simulink library "Enrg_conv_El_to_Mec_zfCetrax"  (R2016a)
settings: Solver=ode1  StartTime=0.0  StopTime=Inf  FixedStep=0.001  RelTol=1e-3
undefined symbols (not defined in the file): drvEmot_RefTqeMOT, FirstDrivenAxle_FirstDrivenAxleNoOfEmot, FirstDrivenAxleNoOfEmot, FMIKit, mec_fRollCoeffOverall, mec_iDiffAxle, mec_massVehicle_kg, mec_rWheelDriven, RefTqeMOT, SecondDrivenAxle_SecondDrivenAxleNoOfEmot, SecondDrivenAxleNoOfEmot
libraries: simulink_extras x3, Enrg_conv_El_to_Mec_zfCetrax x3
(part 3 of 3)

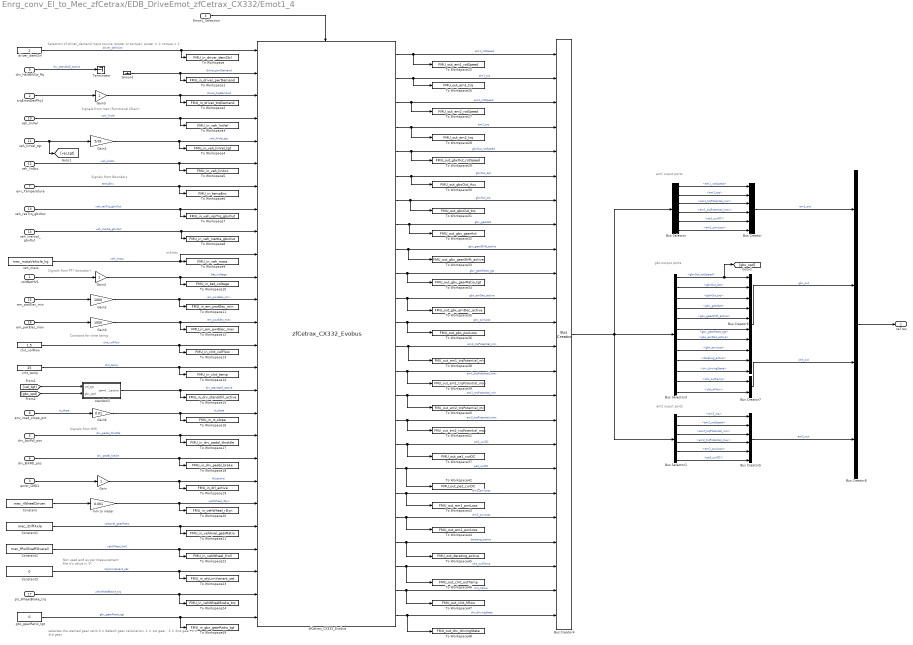
== system Enrg_conv_El_to_Mec_zfCetrax/EDB_DriveEmot_zfCetrax_CX332/Emot1_4 ==
  note: em1 ouput ports
  note: Selection of driver_demand input source (power or torque). power = 1; torque = 2
  note: Signals from Boundary
  note: Signals from HMI
  note: Signals from mec (Functional Chain)
  note: Constant for time being
  note: Signals from PTI (actuator)
  note: em2 ouput ports
  note: gbx output ports
  note: Not used and as per
      | measurement file it's value is '0'
  note: m3/sec
  note: selectes the wanted gear ratio
      | 0 = default gear calculation, 1 = 1st gear , 2 = 2nd gear, 3 = 3rd gear
  voltBatHV1 : Inport
  trqEmotDesPhy1 : Inport  Port=2
  emot_CMD1 : Inport  Port=3
  Emot1_Selection : Inport  Port=4
  drv_AccPdl_pos : Inport  Port=5
  drv_BrkPdl_pos : Inport  Port=6
  env_Temperature : Inport  Port=7
  env_road_slope_pct : Inport  Port=8
  drv_HaltBrkSw_Rq : Inport  Port=9
  veh_linVel : Inport  Port=10
  veh_linVel_tgt : Inport  Port=11
  veh_linAcc : Inport  Port=12
  veh_resTrq_gbxOut : Inport  Port=13
  veh_inertial_gbxOut : Inport  Port=14
  em_pwrElec_min : Inport  Port=15
  em_pwrElec_max : Inport  Port=16
  pti_WheelBrake_trq : Inport  Port=17
  Bus Creator : BusCreator  Inputs=6
  Bus Creator4 : BusCreator  Inputs=24
  Bus Creator5 : BusCreator  Inputs=6
  Bus Creator6 : BusCreator  Inputs=10
  Bus Creator7 : BusCreator  Inputs=2
  Bus Creator8 : BusCreator  Inputs=4
  Bus Selector : BusSelector  OutputSignals=em1_rotSpeed,em1_trq,em1_trqPotential_min,em1_trqPotential_max,pe1_curDC,em1_pwrLoss
  Bus Selector1 : BusSelector  OutputSignals=em2_trq,em2_rotSpeed,em2_trqPotential_min,em2_trqPotential_max,em2_pwrLoss,pe2_curDC
  Bus Selector3 : BusSelector  OutputSignals=gbxOut_rotSpeed,gbxOut_Acc,gbxOut_trq,gbx_gearAct,gbx_gearShift_active,gbx_gearRatio_tgt,gbx_emDec_active,gbx_pwrLoss,derating_active,drv_drivingState,clnt_outTemp,clnt_hFlow
  Constant : Constant  Value=mec_rWheelDriven
  Constant1 : Constant  Value=mec_iDiffAxle
  Constant2 : Constant  Value=mec_fRollCoeffOverall
  Constant3 : Constant  Value=0
  Gain : Gain
  Gain1 : Gain  Gain=5/18
  Gain2 : Gain  Gain=1000
  Gain3 : Gain  Gain=1000
  Gain4 : Gain
  Gain5 : Gain
  Gain6 : Gain  Gain=0.01
  Ground : Ground
  Terminator : Terminator
  To Workspace : ToWorkspace  VariableName=FMU_in_driver_demCtrl  SampleTime=-1
      settings: Save2DSignal=2-D array (concatenate along first dimension)
  To Workspace1 : ToWorkspace  VariableName=FMU_in_driver_pwrDemand  SampleTime=-1
      settings: Save2DSignal=2-D array (concatenate along first dimension)
  To Workspace10 : ToWorkspace  VariableName=FMU_in_bat_voltage  SampleTime=-1
      settings: Save2DSignal=2-D array (concatenate along first dimension)
  To Workspace11 : ToWorkspace  VariableName=FMU_in_em_pwrElec_min  SampleTime=-1
      settings: Save2DSignal=2-D array (concatenate along first dimension)
  To Workspace12 : ToWorkspace  VariableName=FMU_in_em_pwrElec_max  SampleTime=-1
      settings: Save2DSignal=2-D array (concatenate along first dimension)
  To Workspace13 : ToWorkspace  VariableName=FMU_in_clnt_volFlow  SampleTime=-1
      settings: Save2DSignal=2-D array (concatenate along first dimension)
  To Workspace14 : ToWorkspace  VariableName=FMU_in_clnt_temp  SampleTime=-1
      settings: Save2DSignal=2-D array (concatenate along first dimension)
  To Workspace15 : ToWorkspace  VariableName=FMU_in_drv_standstill_active  SampleTime=-1
      settings: Save2DSignal=2-D array (concatenate along first dimension)
  To Workspace16 : ToWorkspace  VariableName=FMU_in_rt_slope  SampleTime=-1
      settings: Save2DSignal=2-D array (concatenate along first dimension)
  To Workspace17 : ToWorkspace  VariableName=FMU_in_drv_pedal_throttle  SampleTime=-1
      settings: Save2DSignal=2-D array (concatenate along first dimension)
  To Workspace18 : ToWorkspace  VariableName=FMU_in_drv_pedal_brake  SampleTime=-1
      settings: Save2DSignal=2-D array (concatenate along first dimension)
  To Workspace19 : ToWorkspace  VariableName=FMU_in_drl_active  SampleTime=-1
      settings: Save2DSignal=2-D array (concatenate along first dimension)
  To Workspace2 : ToWorkspace  VariableName=FMU_in_driver_trqDemand  SampleTime=-1
      settings: Save2DSignal=2-D array (concatenate along first dimension)
  To Workspace20 : ToWorkspace  VariableName=FMU_in_vehWheel_rDyn  SampleTime=-1
      settings: Save2DSignal=2-D array (concatenate along first dimension)
  To Workspace21 : ToWorkspace  VariableName=FMU_in_vehAxel_gearRatio  SampleTime=-1
      settings: Save2DSignal=2-D array (concatenate along first dimension)
  To Workspace22 : ToWorkspace  VariableName=FMU_in_vehWheel_froll  SampleTime=-1
      settings: Save2DSignal=2-D array (concatenate along first dimension)
  To Workspace23 : ToWorkspace  VariableName=FMU_in_styLimVariant_set  SampleTime=-1
      settings: Save2DSignal=2-D array (concatenate along first dimension)
  To Workspace24 : ToWorkspace  VariableName=FMU_in_vehWheelBrake_trq  SampleTime=-1
      settings: Save2DSignal=2-D array (concatenate along first dimension)
  To Workspace25 : ToWorkspace  VariableName=FMU_out_em1_rotSpeed  SampleTime=-1
      settings: Save2DSignal=2-D array (concatenate along first dimension)
  To Workspace26 : ToWorkspace  VariableName=FMU_out_em1_trq  SampleTime=-1
      settings: Save2DSignal=2-D array (concatenate along first dimension)
  To Workspace27 : ToWorkspace  VariableName=FMU_out_em2_rotSpeed  SampleTime=-1
      settings: Save2DSignal=2-D array (concatenate along first dimension)
  To Workspace28 : ToWorkspace  VariableName=FMU_out_em2_trq  SampleTime=-1
      settings: Save2DSignal=2-D array (concatenate along first dimension)
  To Workspace29 : ToWorkspace  VariableName=FMU_out_gbxOut_rotSpeed  SampleTime=-1
      settings: Save2DSignal=2-D array (concatenate along first dimension)
  To Workspace3 : ToWorkspace  VariableName=FMU_in_veh_linVel  SampleTime=-1
      settings: Save2DSignal=2-D array (concatenate along first dimension)
  To Workspace30 : ToWorkspace  VariableName=FMU_out_gbxOut_Acc  SampleTime=-1
      settings: Save2DSignal=2-D array (concatenate along first dimension)
  To Workspace31 : ToWorkspace  VariableName=FMU_out_gbxOut_trq  SampleTime=-1
      settings: Save2DSignal=2-D array (concatenate along first dimension)
  To Workspace32 : ToWorkspace  VariableName=FMU_out_gbx_gearAct  SampleTime=-1
      settings: Save2DSignal=2-D array (concatenate along first dimension)
  To Workspace33 : ToWorkspace  VariableName=FMU_out_gbx_gearShift_active  SampleTime=-1
      settings: Save2DSignal=2-D array (concatenate along first dimension)
  To Workspace34 : ToWorkspace  VariableName=FMU_out_gbx_gearRatio_tgt  SampleTime=-1
      settings: Save2DSignal=2-D array (concatenate along first dimension)
  To Workspace35 : ToWorkspace  VariableName=FMU_out_gbx_emDec_active  SampleTime=-1
      settings: Save2DSignal=2-D array (concatenate along first dimension)
  To Workspace36 : ToWorkspace  VariableName=FMU_out_gbx_pwrLoss  SampleTime=-1
      settings: Save2DSignal=2-D array (concatenate along first dimension)
  To Workspace37 : ToWorkspace  VariableName=FMU_out_pe1_curDC  SampleTime=-1
      settings: Save2DSignal=2-D array (concatenate along first dimension)
  To Workspace38 : ToWorkspace  VariableName=FMU_out_em1_trqPotential_min  SampleTime=-1
      settings: Save2DSignal=2-D array (concatenate along first dimension)
  To Workspace39 : ToWorkspace  VariableName=FMU_out_em1_trqPotential_max  SampleTime=-1
      settings: Save2DSignal=2-D array (concatenate along first dimension)
  To Workspace4 : ToWorkspace  VariableName=FMU_in_veh_linVel_tgt  SampleTime=-1
      settings: Save2DSignal=2-D array (concatenate along first dimension)
  To Workspace40 : ToWorkspace  VariableName=FMU_out_em2_trqPotential_min  SampleTime=-1
      settings: Save2DSignal=2-D array (concatenate along first dimension)
  To Workspace41 : ToWorkspace  VariableName=FMU_out_em2_trqPotential_max  SampleTime=-1
      settings: Save2DSignal=2-D array (concatenate along first dimension)
  To Workspace42 : ToWorkspace  VariableName=FMU_out_pe2_curDC  SampleTime=-1
      settings: Save2DSignal=2-D array (concatenate along first dimension)
  To Workspace43 : ToWorkspace  VariableName=FMU_out_em1_pwrLoss  SampleTime=-1
      settings: Save2DSignal=2-D array (concatenate along first dimension)
  To Workspace44 : ToWorkspace  VariableName=FMU_out_em2_pwrLoss  SampleTime=-1
      settings: Save2DSignal=2-D array (concatenate along first dimension)
  To Workspace45 : ToWorkspace  VariableName=FMU_out_derating_active  SampleTime=-1
      settings: Save2DSignal=2-D array (concatenate along first dimension)
  To Workspace46 : ToWorkspace  VariableName=FMU_out_clnt_outTemp  SampleTime=-1
      settings: Save2DSignal=2-D array (concatenate along first dimension)
  To Workspace47 : ToWorkspace  VariableName=FMU_out_clnt_hflow  SampleTime=-1
      settings: Save2DSignal=2-D array (concatenate along first dimension)
  To Workspace48 : ToWorkspace  VariableName=FMU_out_drv_drivingState  SampleTime=-1
      settings: Save2DSignal=2-D array (concatenate along first dimension)
  To Workspace49 : ToWorkspace  VariableName=FMU_in_gbx_gearRatio_tgt  SampleTime=-1
      settings: Save2DSignal=2-D array (concatenate along first dimension)
  To Workspace5 : ToWorkspace  VariableName=FMU_in_veh_linAcc  SampleTime=-1
      settings: Save2DSignal=2-D array (concatenate along first dimension)
  To Workspace6 : ToWorkspace  VariableName=FMU_in_tempEnv  SampleTime=-1
      settings: Save2DSignal=2-D array (concatenate along first dimension)
  To Workspace7 : ToWorkspace  VariableName=FMU_in_veh_resTrq_gbxOut  SampleTime=-1
      settings: Save2DSignal=2-D array (concatenate along first dimension)
  To Workspace8 : ToWorkspace  VariableName=FMU_in_veh_inertia_gbxOut  SampleTime=-1
      settings: Save2DSignal=2-D array (concatenate along first dimension)
  To Workspace9 : ToWorkspace  VariableName=FMU_in_veh_mass  SampleTime=-1
      settings: Save2DSignal=2-D array (concatenate along first dimension)
  clnt_temp : Constant  Value=25
  clnt_volFlow : Constant  Value=1.5
  driver_demCtrl : Constant  Value=2
  gbx_gearRatio_tgt : Constant  Value=0
  mm to meter : Gain  Gain=0.001
  standstill : Subsystem
  veh_mass : Constant  Value=mec_massVehicle_kg
  zfCetrax_CX332_Evobus : Enrg_conv_El_to_Mec_zfCetrax/zfCetrax_CX332_Evobus  SystemSampleTime=-1
  ceTrax : Outport
  wires:
  zfCetrax_CX332_Evobus/24 -> Bus Creator4/24, To Workspace48/1  "drv_drivingState"
  gbx_gearRatio_tgt/1 -> zfCetrax_CX332_Evobus/26, To Workspace49/1  "gbx_gearRatio_tgt"
  Constant2/1 -> zfCetrax_CX332_Evobus/23, To Workspace22/1  "vehWheel_froll"
  Constant1/1 -> zfCetrax_CX332_Evobus/22, To Workspace21/1  "vehAxel_gearRatio"
  Constant/1 -> mm to meter/1
  emot_CMD1/1 -> Gain/1
  trqEmotDesPhy1/1 -> Gain5/1
  voltBatHV1/1 -> Gain4/1
  Emot1_Selection/1 -> zfCetrax_CX332_Evobus/Enable
  Ground/1 -> zfCetrax_CX332_Evobus/2, To Workspace1/1  "driver_pwrDemand"
  driver_demCtrl/1 -> zfCetrax_CX332_Evobus/1, To Workspace/1  "driver_demCtrl"
  drv_AccPdl_pos/1 -> zfCetrax_CX332_Evobus/18, To Workspace17/1  "drv_pedal_throttle"
  drv_BrkPdl_pos/1 -> zfCetrax_CX332_Evobus/19, To Workspace18/1  "drv_pedal_brake"
  env_Temperature/1 -> zfCetrax_CX332_Evobus/7, To Workspace6/1  "tempEnv"
  env_road_slope_pct/1 -> Gain6/1  "rt_slope"
  veh_mass/1 -> zfCetrax_CX332_Evobus/10, To Workspace9/1  "veh_mass"
  veh_linVel/1 -> zfCetrax_CX332_Evobus/4, To Workspace3/1  "veh_linVel"
  veh_linVel_tgt/1 -> Gain1/1, [vel_tgt]
  veh_linAcc/1 -> zfCetrax_CX332_Evobus/6, To Workspace5/1  "veh_linAcc"
  veh_inertial_gbxOut/1 -> zfCetrax_CX332_Evobus/9, To Workspace8/1  "veh_inertia_gbxOut"
  clnt_temp/1 -> zfCetrax_CX332_Evobus/15, To Workspace14/1  "clnt_temp"
  clnt_volFlow/1 -> zfCetrax_CX332_Evobus/14, To Workspace13/1  "clnt_volFlow"
  em_pwrElec_max/1 -> Gain3/1
  em_pwrElec_min/1 -> Gain2/1
  zfCetrax_CX332_Evobus/8 -> To Workspace32/1, Bus Creator4/8  "gbx_gearAct"
  zfCetrax_CX332_Evobus/10 -> To Workspace34/1, Bus Creator4/10  "gbx_gearRatio_tgt"
  zfCetrax_CX332_Evobus/4 -> To Workspace28/1, Bus Creator4/4  "em2_trq"
  zfCetrax_CX332_Evobus/11 -> To Workspace35/1, Bus Creator4/11  "gbx_emDec_active"
  zfCetrax_CX332_Evobus/12 -> To Workspace36/1, Bus Creator4/12  "gbx_pwrLoss"
  zfCetrax_CX332_Evobus/13 -> To Workspace38/1, Bus Creator4/13  "em1_trqPotential_min"
  zfCetrax_CX332_Evobus/15 -> To Workspace40/1, Bus Creator4/15  "em2_trqPotential_min"
  zfCetrax_CX332_Evobus/9 -> To Workspace33/1, Bus Creator4/9  "gbx_gearShift_active"
  zfCetrax_CX332_Evobus/7 -> To Workspace31/1, Bus Creator4/7  "gbxOut_trq"
  zfCetrax_CX332_Evobus/17 -> To Workspace37/1, Bus Creator4/17  "pe1_curDC"
  zfCetrax_CX332_Evobus/14 -> To Workspace39/1, Bus Creator4/14  "em1_trqPotential_max"
  zfCetrax_CX332_Evobus/1 -> To Workspace25/1, Bus Creator4/1  "em1_rotSpeed"
  zfCetrax_CX332_Evobus/6 -> To Workspace30/1, Bus Creator4/6  "gbxOut_Acc"
  zfCetrax_CX332_Evobus/16 -> To Workspace41/1, Bus Creator4/16  "em2_trqPotential_max"
  zfCetrax_CX332_Evobus/18 -> To Workspace42/1, Bus Creator4/18  "pe2_curDC"
  zfCetrax_CX332_Evobus/2 -> To Workspace26/1, Bus Creator4/2  "em1_trq"
  zfCetrax_CX332_Evobus/3 -> To Workspace27/1, Bus Creator4/3  "em2_rotSpeed"
  zfCetrax_CX332_Evobus/5 -> To Workspace29/1, Bus Creator4/5  "gbxOut_rotSpeed"
  zfCetrax_CX332_Evobus/20 -> To Workspace44/1, Bus Creator4/20  "em2_pwrLoss"
  zfCetrax_CX332_Evobus/19 -> To Workspace43/1, Bus Creator4/19  "em1_pwrLoss"
  zfCetrax_CX332_Evobus/21 -> To Workspace45/1, Bus Creator4/21  "derating_active"
  zfCetrax_CX332_Evobus/23 -> To Workspace47/1, Bus Creator4/23  "clnt_hFlow"
  zfCetrax_CX332_Evobus/22 -> To Workspace46/1, Bus Creator4/22  "clnt_outTemp"
  Bus Creator4/1 -> Bus Selector1/1, Bus Selector3/1, Bus Selector/1
  Gain1/1 -> zfCetrax_CX332_Evobus/5, To Workspace4/1  "veh_linVel_tgt"
  Bus Selector/1 -> Bus Creator/1  "<em1_rotSpeed>"
  Bus Selector/2 -> Bus Creator/2  "<em1_trq>"
  Bus Selector/3 -> Bus Creator/3  "<em1_trqPotential_min>"
  Bus Selector/4 -> Bus Creator/4  "<em1_trqPotential_max>"
  Bus Selector/5 -> Bus Creator/5  "<pe1_curDC>"
  Bus Selector/6 -> Bus Creator/6  "<em1_pwrLoss>"
  Bus Selector1/1 -> Bus Creator5/1  "<em2_trq>"
  Bus Selector1/2 -> Bus Creator5/2  "<em2_rotSpeed>"
  Bus Selector1/3 -> Bus Creator5/3  "<em2_trqPotential_min>"
  Bus Selector1/4 -> Bus Creator5/4  "<em2_trqPotential_max>"
  Bus Selector1/5 -> Bus Creator5/5  "<em2_pwrLoss>"
  Bus Selector1/6 -> Bus Creator5/6  "<pe2_curDC>"
  Bus Selector3/1 -> [gbx_spd], Bus Creator6/1  "<gbxOut_rotSpeed>"
  Bus Selector3/2 -> Bus Creator6/2  "<gbxOut_Acc>"
  Bus Selector3/3 -> Bus Creator6/3  "<gbxOut_trq>"
  Bus Selector3/4 -> Bus Creator6/4  "<gbx_gearAct>"
  Bus Selector3/5 -> Bus Creator6/5  "<gbx_gearShift_active>"
  Bus Selector3/6 -> Bus Creator6/6  "<gbx_gearRatio_tgt>"
  Bus Selector3/7 -> Bus Creator6/7  "<gbx_emDec_active>"
  Bus Selector3/8 -> Bus Creator6/8  "<gbx_pwrLoss>"
  Bus Selector3/9 -> Bus Creator6/9  "<derating_active>"
  Bus Selector3/11 -> Bus Creator7/1  "<clnt_outTemp>"
  Bus Selector3/12 -> Bus Creator7/2  "<clnt_hFlow>"
  Bus Creator/1 -> Bus Creator8/1  "em1_out"
  Bus Creator5/1 -> Bus Creator8/4  "em2_out"
  Bus Creator6/1 -> Bus Creator8/2  "gbx_out"
  Bus Creator7/1 -> Bus Creator8/3  "clnt_out"
  Bus Creator8/1 -> ceTrax/1
  Gain2/1 -> zfCetrax_CX332_Evobus/12, To Workspace11/1  "em_pwrElec_min"
  Gain3/1 -> zfCetrax_CX332_Evobus/13, To Workspace12/1  "em_pwrElec_max"
  mm to meter/1 -> zfCetrax_CX332_Evobus/21, To Workspace20/1  "vehWheel_rDyn"
  Constant3/1 -> zfCetrax_CX332_Evobus/24, To Workspace23/1  "stylLimVariant_set"
  pti_WheelBrake_trq/1 -> zfCetrax_CX332_Evobus/25, To Workspace24/1  "vehWheelBrake_trq"
  standstill/1(standstill_active) -> zfCetrax_CX332_Evobus/16, To Workspace15/1  "drv_standstill_active"
  Gain/1 -> zfCetrax_CX332_Evobus/20, To Workspace19/1  "drl_active"
  Gain4/1 -> zfCetrax_CX332_Evobus/11, To Workspace10/1  "bat_voltage"
  Gain5/1 -> zfCetrax_CX332_Evobus/3, To Workspace2/1  "driver_trqDemand"
  veh_resTrq_gbxOut/1 -> zfCetrax_CX332_Evobus/8, To Workspace7/1  "veh_resTrq_gbxOut"
  Gain6/1 -> zfCetrax_CX332_Evobus/17, To Workspace16/1  "rt_slope"
  drv_HaltBrkSw_Rq/1 -> Terminator/1  "drv_standstill_active"
  [vel_tgt] -> standstill/1(vel_tgt)
  [gbx_spd] -> standstill/2(gbx_spd)
  Bus Selector3/10 -> Bus Creator6/10  "<drv_drivingState>"

== system Enrg_conv_El_to_Mec_zfCetrax/EDB_DriveEmot_zfCetrax_CX332/MotorSelection ==
  MidAxle : Constant  Value=FirstDrivenAxleNoOfEmot
  RearAxle : Constant  Value=SecondDrivenAxleNoOfEmot
  Truth Table : Truth Table  TreatAsAtomicUnit=on
  Emot1_Selection : Outport
  Emot2_Selection : Outport  Port=2
  Emot3_Selection : Outport  Port=3
  Emot4_Selection : Outport  Port=4
  wires:
  MidAxle/1 -> Truth Table/1(u1)
  RearAxle/1 -> Truth Table/2(u2)
  Truth Table/1(y1) -> Emot1_Selection/1
  Truth Table/2(y2) -> Emot2_Selection/1
  Truth Table/3(y3) -> Emot3_Selection/1
  Truth Table/4(y4) -> Emot4_Selection/1

== system Enrg_conv_El_to_Mec_zfCetrax/EDB_DriveEmot_zfCetrax/EMD1_Selection/percent_to_Nm2 ==
  Percentage_Torque : Inport
  Reference_Torque : Inport  Port=2
  Constant : Constant  Value=100
  Divide : Product  Inputs=*/
  Product : Product  RndMeth=Zero
  Torque_Nm : Outport
  wires:
  Percentage_Torque/1 -> Product/1  "Percentage_Torque"
  Divide/1 -> Torque_Nm/1  "Torque_Nm"
  Reference_Torque/1 -> Product/2  "Reference_Torque"
  Product/1 -> Divide/1
  Constant/1 -> Divide/2

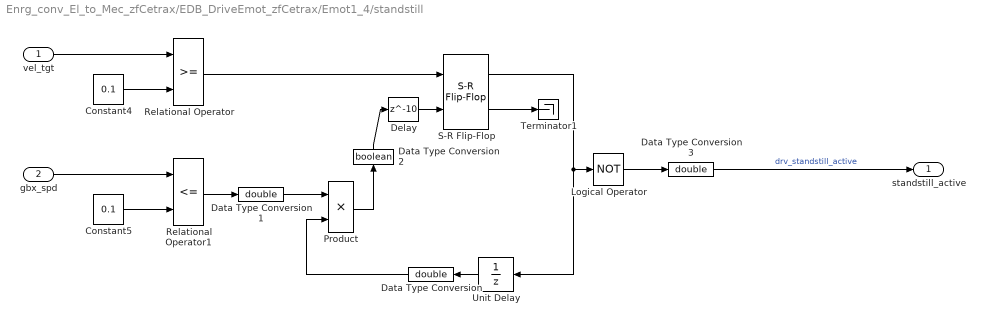
== system Enrg_conv_El_to_Mec_zfCetrax/EDB_DriveEmot_zfCetrax/Emot1_4/standstill ==
  vel_tgt : Inport
  gbx_spd : Inport  Port=2
  Constant4 : Constant  Value=0.1
  Constant5 : Constant  Value=0.1
  Data Type Conversion : DataTypeConversion  OutDataTypeStr=double
  Data Type Conversion1 : DataTypeConversion  OutDataTypeStr=double
  Data Type Conversion2 : DataTypeConversion  OutDataTypeStr=boolean
  Data Type Conversion3 : DataTypeConversion  OutDataTypeStr=double
  Delay : Delay  DelayLength=10
  Logical Operator : Logic  Operator=NOT  AllPortsSameDT=off  OutDataTypeStr=boolean
  Product : Product
  Relational Operator : RelationalOperator  OutDataTypeStr=boolean
  Relational Operator1 : RelationalOperator  Operator=<=  OutDataTypeStr=boolean
  S-R Flip-Flop : simulink_extras/Flip Flops/S-R Flip-Flop  initial_condition=0
  Terminator1 : Terminator
  Unit Delay : UnitDelay  SampleTime=-1
  standstill_active : Outport
  wires:
  gbx_spd/1 -> Relational Operator1/1
  Relational Operator1/1 -> Data Type Conversion1/1
  Delay/1 -> S-R Flip-Flop/2
  Data Type Conversion1/1 -> Product/1
  Constant4/1 -> Relational Operator/2
  Logical Operator/1 -> Data Type Conversion3/1
  vel_tgt/1 -> Relational Operator/1
  Relational Operator/1 -> S-R Flip-Flop/1
  Data Type Conversion/1 -> Product/2
  Constant5/1 -> Relational Operator1/2
  Data Type Conversion3/1 -> standstill_active/1  "drv_standstill_active"
  Data Type Conversion2/1 -> Delay/1
  S-R Flip-Flop/2 -> Terminator1/1
  Product/1 -> Data Type Conversion2/1
  S-R Flip-Flop/1 -> Unit Delay/1, Logical Operator/1
  Unit Delay/1 -> Data Type Conversion/1

== system Enrg_conv_El_to_Mec_zfCetrax/EDB_DriveEmot_zfCetrax_CX319/EMD1_Selection/percent_to_Nm2 ==
  Percentage_Torque : Inport
  Reference_Torque : Inport  Port=2
  Constant : Constant  Value=100
  Divide : Product  Inputs=*/
  Product : Product  RndMeth=Zero
  Torque_Nm : Outport
  wires:
  Constant/1 -> Divide/2
  Product/1 -> Divide/1
  Reference_Torque/1 -> Product/2  "Reference_Torque"
  Divide/1 -> Torque_Nm/1  "Torque_Nm"
  Percentage_Torque/1 -> Product/1  "Percentage_Torque"

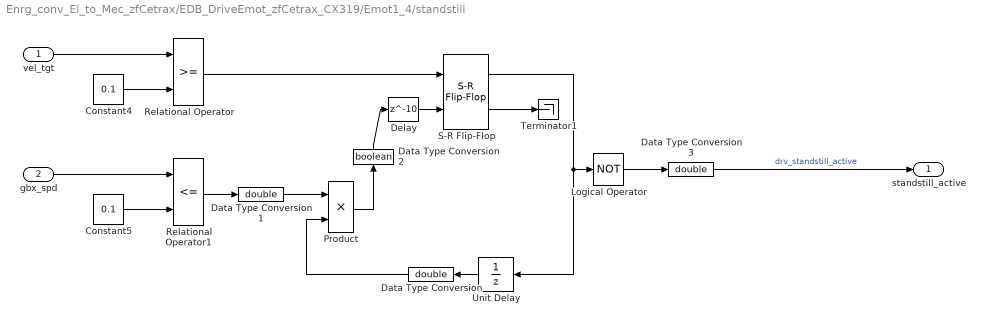
== system Enrg_conv_El_to_Mec_zfCetrax/EDB_DriveEmot_zfCetrax_CX319/Emot1_4/standstill ==
  vel_tgt : Inport
  gbx_spd : Inport  Port=2
  Constant4 : Constant  Value=0.1
  Constant5 : Constant  Value=0.1
  Data Type Conversion : DataTypeConversion  OutDataTypeStr=double
  Data Type Conversion1 : DataTypeConversion  OutDataTypeStr=double
  Data Type Conversion2 : DataTypeConversion  OutDataTypeStr=boolean
  Data Type Conversion3 : DataTypeConversion  OutDataTypeStr=double
  Delay : Delay  DelayLength=10
  Logical Operator : Logic  Operator=NOT  AllPortsSameDT=off  OutDataTypeStr=boolean
  Product : Product
  Relational Operator : RelationalOperator  OutDataTypeStr=boolean
  Relational Operator1 : RelationalOperator  Operator=<=  OutDataTypeStr=boolean
  S-R Flip-Flop : simulink_extras/Flip Flops/S-R Flip-Flop  initial_condition=0
  Terminator1 : Terminator
  Unit Delay : UnitDelay  SampleTime=-1
  standstill_active : Outport
  wires:
  Unit Delay/1 -> Data Type Conversion/1
  S-R Flip-Flop/1 -> Logical Operator/1, Unit Delay/1
  Product/1 -> Data Type Conversion2/1
  S-R Flip-Flop/2 -> Terminator1/1
  Data Type Conversion2/1 -> Delay/1
  Data Type Conversion3/1 -> standstill_active/1  "drv_standstill_active"
  Constant5/1 -> Relational Operator1/2
  Data Type Conversion/1 -> Product/2
  Relational Operator/1 -> S-R Flip-Flop/1
  vel_tgt/1 -> Relational Operator/1
  Logical Operator/1 -> Data Type Conversion3/1
  Constant4/1 -> Relational Operator/2
  Data Type Conversion1/1 -> Product/1
  Delay/1 -> S-R Flip-Flop/2
  Relational Operator1/1 -> Data Type Conversion1/1
  gbx_spd/1 -> Relational Operator1/1

== system Enrg_conv_El_to_Mec_zfCetrax/EDB_DriveEmot_zfCetrax_CX332/EMD1_Selection/percent_to_Nm2 ==
  Percentage_Torque : Inport
  Reference_Torque : Inport  Port=2
  Constant : Constant  Value=100
  Divide : Product  Inputs=*/
  Product : Product  RndMeth=Zero
  Torque_Nm : Outport
  wires:
  Percentage_Torque/1 -> Product/1  "Percentage_Torque"
  Divide/1 -> Torque_Nm/1  "Torque_Nm"
  Reference_Torque/1 -> Product/2  "Reference_Torque"
  Product/1 -> Divide/1
  Constant/1 -> Divide/2

== system Enrg_conv_El_to_Mec_zfCetrax/EDB_DriveEmot_zfCetrax_CX332/Emot1_4/standstill ==
  vel_tgt : Inport
  gbx_spd : Inport  Port=2
  Constant4 : Constant  Value=0.1
  Constant5 : Constant  Value=0.1
  Data Type Conversion : DataTypeConversion  OutDataTypeStr=double
  Data Type Conversion1 : DataTypeConversion  OutDataTypeStr=double
  Data Type Conversion2 : DataTypeConversion  OutDataTypeStr=boolean
  Data Type Conversion3 : DataTypeConversion  OutDataTypeStr=double
  Delay : Delay  DelayLength=10
  Logical Operator : Logic  Operator=NOT  AllPortsSameDT=off  OutDataTypeStr=boolean
  Product : Product
  Relational Operator : RelationalOperator  OutDataTypeStr=boolean
  Relational Operator1 : RelationalOperator  Operator=<=  OutDataTypeStr=boolean
  S-R Flip-Flop : simulink_extras/Flip Flops/S-R Flip-Flop  initial_condition=0
  Terminator1 : Terminator
  Unit Delay : UnitDelay  SampleTime=-1
  standstill_active : Outport
  wires:
  gbx_spd/1 -> Relational Operator1/1
  Relational Operator1/1 -> Data Type Conversion1/1
  Delay/1 -> S-R Flip-Flop/2
  Data Type Conversion1/1 -> Product/1
  Constant4/1 -> Relational Operator/2
  Logical Operator/1 -> Data Type Conversion3/1
  vel_tgt/1 -> Relational Operator/1
  Relational Operator/1 -> S-R Flip-Flop/1
  Data Type Conversion/1 -> Product/2
  Constant5/1 -> Relational Operator1/2
  Data Type Conversion3/1 -> standstill_active/1  "drv_standstill_active"
  Data Type Conversion2/1 -> Delay/1
  S-R Flip-Flop/2 -> Terminator1/1
  Product/1 -> Data Type Conversion2/1
  S-R Flip-Flop/1 -> Unit Delay/1, Logical Operator/1
  Unit Delay/1 -> Data Type Conversion/1

== matlab function Enrg_conv_El_to_Mec_zfCetrax/EDB_DriveEmot_zfCetrax_CX319/MotorSelection/Truth Table ==
  data: u1 input; y1 output; u2 input; y2 output; y3 output; y4 output
function [y1, y2, y3, y4] = fcn(u1, u2)

aVarTruthTableCondition_1 = false;
aVarTruthTableCondition_2 = false;
aVarTruthTableCondition_3 = false;
aVarTruthTableCondition_4 = false;
aVarTruthTableCondition_5 = false;
aVarTruthTableCondition_6 = false;
aVarTruthTableCondition_7 = false;
aVarTruthTableCondition_8 = false;
aVarTruthTableCondition_9 = false;


% 1stDrivenAxle - 0  and 2ndDrivenAxle - 0 [Not Valid]

aVarTruthTableCondition_1 = logical(u1 == 0 && u2 == 0);

% 1stDrivenAxle - 0  and 2ndDrivenAxle - 1 [Not Valid]

aVarTruthTableCondition_2 = logical(u1 == 0 && u2 == 1);

% 1stDrivenAxle - 0  and 2ndDrivenAxle - 2 [Not Valid]

aVarTruthTableCondition_3 = logical(u1 == 0 && u2 == 2);

% 1stDrivenAxle - 1  and 2ndDrivenAxle - 0 [Emot1,-]

aVarTruthTableCondition_4 = logical(u1 == 1 && u2 == 0);

% 1stDrivenAxle - 1  and 2ndDrivenAxle - 1 [Emot1, Emot3]

aVarTruthTableCondition_5 = logical(u1 == 1 && u2 == 1);

% 1stDrivenAxle - 1  and 2ndDrivenAxle - 2 [Emot1, Emot3+Emot4]

aVarTruthTableCondition_6 = logical(u1 == 1 && u2 == 2);

% 1stDrivenAxle - 2  and 2ndDrivenAxle - 0 [Emot1+Emot2,-]

aVarTruthTableCondition_7 = logical(u1 == 2 && u2 == 0);

% 1stDrivenAxle - 2  and 2ndDrivenAxle - 1 [Emot1+Emot2,Emot3]

aVarTruthTableCondition_8 = logical(u1 == 2 && u2 == 1);

% 1stDrivenAxle - 2  and2ndDrivenAxle - 2 [Emot1+Emot2,Emot3+Emot4]

aVarTruthTableCondition_9 = logical(u1 == 2 && u2 == 2);

if (aVarTruthTableCondition_1 && ~aVarTruthTableCondition_2 && ~aVarTruthTableCondition_3 && ~aVarTruthTableCondition_4 && ~aVarTruthTableCondition_5 && ~aVarTruthTableCondition_6 && ~aVarTruthTableCondition_7 && ~aVarTruthTableCondition_8 && ~aVarTruthTableCondition_9)
    aFcnTruthTableAction_1();
elseif (~aVarTruthTableCondition_1 && aVarTruthTableCondition_2 && ~aVarTruthTableCondition_3 && ~aVarTruthTableCondition_4 && ~aVarTruthTableCondition_5 && ~aVarTruthTableCondition_6 && ~aVarTruthTableCondition_7 && ~aVarTruthTableCondition_8 && ~aVarTruthTableCondition_9)
    aFcnTruthTableAction_2();
elseif (~aVarTruthTableCondition_1 && ~aVarTruthTableCondition_2 && aVarTruthTableCondition_3 && ~aVarTruthTableCondition_4 && ~aVarTruthTableCondition_5 && ~aVarTruthTableCondition_6 && ~aVarTruthTableCondition_7 && ~aVarTruthTableCondition_8 && ~aVarTruthTableCondition_9)
    aFcnTruthTableAction_3();
elseif (~aVarTruthTableCondition_1 && ~aVarTruthTableCondition_2 && ~aVarTruthTableCondition_3 && aVarTruthTableCondition_4 && ~aVarTruthTableCondition_5 && ~aVarTruthTableCondition_6 && ~aVarTruthTableCondition_7 && ~aVarTruthTableCondition_8 && ~aVarTruthTableCondition_9)
    aFcnTruthTableAction_4();
elseif (~aVarTruthTableCondition_1 && ~aVarTruthTableCondition_2 && ~aVarTruthTableCondition_3 && ~aVarTruthTableCondition_4 && aVarTruthTableCondition_5 && ~aVarTruthTableCondition_6 && ~aVarTruthTableCondition_7 && ~aVarTruthTableCondition_8 && ~aVarTruthTableCondition_9)
    aFcnTruthTableAction_5();
elseif (~aVarTruthTableCondition_1 && ~aVarTruthTableCondition_2 && ~aVarTruthTableCondition_3 && ~aVarTruthTableCondition_4 && ~aVarTruthTableCondition_5 && aVarTruthTableCondition_6 && ~aVarTruthTableCondition_7 && ~aVarTruthTableCondition_8 && ~aVarTruthTableCondition_9)
    aFcnTruthTableAction_6();
elseif (~aVarTruthTableCondition_1 && ~aVarTruthTableCondition_2 && ~aVarTruthTableCondition_3 && ~aVarTruthTableCondition_4 && ~aVarTruthTableCondition_5 && ~aVarTruthTableCondition_6 && aVarTruthTableCondition_7 && ~aVarTruthTableCondition_8 && ~aVarTruthTableCondition_9)
    aFcnTruthTableAction_7();
elseif (~aVarTruthTableCondition_1 && ~aVarTruthTableCondition_2 && ~aVarTruthTableCondition_3 && ~aVarTruthTableCondition_4 && ~aVarTruthTableCondition_5 && ~aVarTruthTableCondition_6 && ~aVarTruthTableCondition_7 && aVarTruthTableCondition_8 && ~aVarTruthTableCondition_9)
    aFcnTruthTableAction_8();
elseif (~aVarTruthTableCondition_1 && ~aVarTruthTableCondition_2 && ~aVarTruthTableCondition_3 && ~aVarTruthTableCondition_4 && ~aVarTruthTableCondition_5 && ~aVarTruthTableCondition_6 && ~aVarTruthTableCondition_7 && ~aVarTruthTableCondition_8 && aVarTruthTableCondition_9)
    aFcnTruthTableAction_9();
else % Default
    aFcnTruthTableAction_10();
end

function aFcnTruthTableAction_1()

% 1stDrivenAxle - 0 
% 2ndDrivenAxle - 0
% NOT VALID

y1 = 0;
y2 = 0;
y3 = 0;
y4 = 0;

function aFcnTruthTableAction_2()

% 1stDrivenAxle - 0 
% 2ndDrivenAxle - 1
% NOT VALID

y1 = 0;
y2 = 0;
y3 = 0;
y4 = 0;

function aFcnTruthTableAction_3()

% 1stDrivenAxle - 0 
% 2ndDrivenAxle - 2
% NOT VALID

y1 = 0;
y2 = 0;
y3 = 0;
y4 = 0;

function aFcnTruthTableAction_4()

% 1stDrivenAxle - 1 
% 2ndDrivenAxle - 0 [Emot1,-]

y1 = 1;
y2 = 0;
y3 = 0;
y4 = 0;

function aFcnTruthTableAction_5()

% 1stDrivenAxle - 1  
% 2ndDrivenAxle - 1 [Emot1, Emot3]

y1 = 1;
y2 = 0;
y3 = 1;
y4 = 0;

function aFcnTruthTableAction_6()

% 1stDrivenAxle - 1 
% 2ndDrivenAxle - 2 [Emot1, Emot3+Emot4]

y1 = 1;
y2 = 0;
y3 = 1;
y4 = 1;

function aFcnTruthTableAction_7()

% 1stDrivenAxle - 2  
% 2ndDrivenAxle - 0 [Emot1+Emot2,-]

y1 = 1;
y2 = 1;
y3 = 0;
y4 = 0;

function aFcnTruthTableAction_8()

% 1stDrivenAxle - 2  
% 2ndDrivenAxle - 1 [Emot1+Emot2,Emot3]

y1 = 1;
y2 = 1;
y3 = 1;
y4 = 0;

function aFcnTruthTableAction_9()

% 1stDrivenAxle - 2
% 2ndDrivenAxle - 2 [Emot1+Emot2,Emot3+Emot4]

y1 = 1;
y2 = 1;
y3 = 1;
y4 = 1;

function aFcnTruthTableAction_10()

% Default

y1 = 0;
y2 = 0;
y3 = 0;
y4 = 0;

== matlab function Enrg_conv_El_to_Mec_zfCetrax/EDB_DriveEmot_zfCetrax/MotorSelection/Truth Table ==
  data: u1 input; y1 output; u2 input; y2 output; y3 output; y4 output
function [y1, y2, y3, y4] = fcn(u1, u2)

aVarTruthTableCondition_1 = false;
aVarTruthTableCondition_2 = false;
aVarTruthTableCondition_3 = false;
aVarTruthTableCondition_4 = false;
aVarTruthTableCondition_5 = false;
aVarTruthTableCondition_6 = false;
aVarTruthTableCondition_7 = false;
aVarTruthTableCondition_8 = false;
aVarTruthTableCondition_9 = false;


% 1stDrivenAxle - 0  and 2ndDrivenAxle - 0 [Not Valid]

aVarTruthTableCondition_1 = logical(u1 == 0 && u2 == 0);

% 1stDrivenAxle - 0  and 2ndDrivenAxle - 1 [Not Valid]

aVarTruthTableCondition_2 = logical(u1 == 0 && u2 == 1);

% 1stDrivenAxle - 0  and 2ndDrivenAxle - 2 [Not Valid]

aVarTruthTableCondition_3 = logical(u1 == 0 && u2 == 2);

% 1stDrivenAxle - 1  and 2ndDrivenAxle - 0 [Emot1,-]

aVarTruthTableCondition_4 = logical(u1 == 1 && u2 == 0);

% 1stDrivenAxle - 1  and 2ndDrivenAxle - 1 [Emot1, Emot3]

aVarTruthTableCondition_5 = logical(u1 == 1 && u2 == 1);

% 1stDrivenAxle - 1  and 2ndDrivenAxle - 2 [Emot1, Emot3+Emot4]

aVarTruthTableCondition_6 = logical(u1 == 1 && u2 == 2);

% 1stDrivenAxle - 2  and 2ndDrivenAxle - 0 [Emot1+Emot2,-]

aVarTruthTableCondition_7 = logical(u1 == 2 && u2 == 0);

% 1stDrivenAxle - 2  and 2ndDrivenAxle - 1 [Emot1+Emot2,Emot3]

aVarTruthTableCondition_8 = logical(u1 == 2 && u2 == 1);

% 1stDrivenAxle - 2  and2ndDrivenAxle - 2 [Emot1+Emot2,Emot3+Emot4]

aVarTruthTableCondition_9 = logical(u1 == 2 && u2 == 2);

if (aVarTruthTableCondition_1 && ~aVarTruthTableCondition_2 && ~aVarTruthTableCondition_3 && ~aVarTruthTableCondition_4 && ~aVarTruthTableCondition_5 && ~aVarTruthTableCondition_6 && ~aVarTruthTableCondition_7 && ~aVarTruthTableCondition_8 && ~aVarTruthTableCondition_9)
    aFcnTruthTableAction_1();
elseif (~aVarTruthTableCondition_1 && aVarTruthTableCondition_2 && ~aVarTruthTableCondition_3 && ~aVarTruthTableCondition_4 && ~aVarTruthTableCondition_5 && ~aVarTruthTableCondition_6 && ~aVarTruthTableCondition_7 && ~aVarTruthTableCondition_8 && ~aVarTruthTableCondition_9)
    aFcnTruthTableAction_2();
elseif (~aVarTruthTableCondition_1 && ~aVarTruthTableCondition_2 && aVarTruthTableCondition_3 && ~aVarTruthTableCondition_4 && ~aVarTruthTableCondition_5 && ~aVarTruthTableCondition_6 && ~aVarTruthTableCondition_7 && ~aVarTruthTableCondition_8 && ~aVarTruthTableCondition_9)
    aFcnTruthTableAction_3();
elseif (~aVarTruthTableCondition_1 && ~aVarTruthTableCondition_2 && ~aVarTruthTableCondition_3 && aVarTruthTableCondition_4 && ~aVarTruthTableCondition_5 && ~aVarTruthTableCondition_6 && ~aVarTruthTableCondition_7 && ~aVarTruthTableCondition_8 && ~aVarTruthTableCondition_9)
    aFcnTruthTableAction_4();
elseif (~aVarTruthTableCondition_1 && ~aVarTruthTableCondition_2 && ~aVarTruthTableCondition_3 && ~aVarTruthTableCondition_4 && aVarTruthTableCondition_5 && ~aVarTruthTableCondition_6 && ~aVarTruthTableCondition_7 && ~aVarTruthTableCondition_8 && ~aVarTruthTableCondition_9)
    aFcnTruthTableAction_5();
elseif (~aVarTruthTableCondition_1 && ~aVarTruthTableCondition_2 && ~aVarTruthTableCondition_3 && ~aVarTruthTableCondition_4 && ~aVarTruthTableCondition_5 && aVarTruthTableCondition_6 && ~aVarTruthTableCondition_7 && ~aVarTruthTableCondition_8 && ~aVarTruthTableCondition_9)
    aFcnTruthTableAction_6();
elseif (~aVarTruthTableCondition_1 && ~aVarTruthTableCondition_2 && ~aVarTruthTableCondition_3 && ~aVarTruthTableCondition_4 && ~aVarTruthTableCondition_5 && ~aVarTruthTableCondition_6 && aVarTruthTableCondition_7 && ~aVarTruthTableCondition_8 && ~aVarTruthTableCondition_9)
    aFcnTruthTableAction_7();
elseif (~aVarTruthTableCondition_1 && ~aVarTruthTableCondition_2 && ~aVarTruthTableCondition_3 && ~aVarTruthTableCondition_4 && ~aVarTruthTableCondition_5 && ~aVarTruthTableCondition_6 && ~aVarTruthTableCondition_7 && aVarTruthTableCondition_8 && ~aVarTruthTableCondition_9)
    aFcnTruthTableAction_8();
elseif (~aVarTruthTableCondition_1 && ~aVarTruthTableCondition_2 && ~aVarTruthTableCondition_3 && ~aVarTruthTableCondition_4 && ~aVarTruthTableCondition_5 && ~aVarTruthTableCondition_6 && ~aVarTruthTableCondition_7 && ~aVarTruthTableCondition_8 && aVarTruthTableCondition_9)
    aFcnTruthTableAction_9();
else % Default
    aFcnTruthTableAction_10();
end

function aFcnTruthTableAction_1()

% 1stDrivenAxle - 0 
% 2ndDrivenAxle - 0
% NOT VALID

y1 = 0;
y2 = 0;
y3 = 0;
y4 = 0;

function aFcnTruthTableAction_2()

% 1stDrivenAxle - 0 
% 2ndDrivenAxle - 1
% NOT VALID

y1 = 0;
y2 = 0;
y3 = 0;
y4 = 0;

function aFcnTruthTableAction_3()

% 1stDrivenAxle - 0 
% 2ndDrivenAxle - 2
% NOT VALID

y1 = 0;
y2 = 0;
y3 = 0;
y4 = 0;

function aFcnTruthTableAction_4()

% 1stDrivenAxle - 1 
% 2ndDrivenAxle - 0 [Emot1,-]

y1 = 1;
y2 = 0;
y3 = 0;
y4 = 0;

function aFcnTruthTableAction_5()

% 1stDrivenAxle - 1  
% 2ndDrivenAxle - 1 [Emot1, Emot3]

y1 = 1;
y2 = 0;
y3 = 1;
y4 = 0;

function aFcnTruthTableAction_6()

% 1stDrivenAxle - 1 
% 2ndDrivenAxle - 2 [Emot1, Emot3+Emot4]

y1 = 1;
y2 = 0;
y3 = 1;
y4 = 1;

function aFcnTruthTableAction_7()

% 1stDrivenAxle - 2  
% 2ndDrivenAxle - 0 [Emot1+Emot2,-]

y1 = 1;
y2 = 1;
y3 = 0;
y4 = 0;

function aFcnTruthTableAction_8()

% 1stDrivenAxle - 2  
% 2ndDrivenAxle - 1 [Emot1+Emot2,Emot3]

y1 = 1;
y2 = 1;
y3 = 1;
y4 = 0;

function aFcnTruthTableAction_9()

% 1stDrivenAxle - 2
% 2ndDrivenAxle - 2 [Emot1+Emot2,Emot3+Emot4]

y1 = 1;
y2 = 1;
y3 = 1;
y4 = 1;

function aFcnTruthTableAction_10()

% Default

y1 = 0;
y2 = 0;
y3 = 0;
y4 = 0;

== matlab function Enrg_conv_El_to_Mec_zfCetrax/EDB_DriveEmot_zfCetrax_CX332/MotorSelection/Truth Table ==
  data: u1 input; y1 output; u2 input; y2 output; y3 output; y4 output
function [y1, y2, y3, y4] = fcn(u1, u2)

aVarTruthTableCondition_1 = false;
aVarTruthTableCondition_2 = false;
aVarTruthTableCondition_3 = false;
aVarTruthTableCondition_4 = false;
aVarTruthTableCondition_5 = false;
aVarTruthTableCondition_6 = false;
aVarTruthTableCondition_7 = false;
aVarTruthTableCondition_8 = false;
aVarTruthTableCondition_9 = false;


% 1stDrivenAxle - 0  and 2ndDrivenAxle - 0 [Not Valid]

aVarTruthTableCondition_1 = logical(u1 == 0 && u2 == 0);

% 1stDrivenAxle - 0  and 2ndDrivenAxle - 1 [Not Valid]

aVarTruthTableCondition_2 = logical(u1 == 0 && u2 == 1);

% 1stDrivenAxle - 0  and 2ndDrivenAxle - 2 [Not Valid]

aVarTruthTableCondition_3 = logical(u1 == 0 && u2 == 2);

% 1stDrivenAxle - 1  and 2ndDrivenAxle - 0 [Emot1,-]

aVarTruthTableCondition_4 = logical(u1 == 1 && u2 == 0);

% 1stDrivenAxle - 1  and 2ndDrivenAxle - 1 [Emot1, Emot3]

aVarTruthTableCondition_5 = logical(u1 == 1 && u2 == 1);

% 1stDrivenAxle - 1  and 2ndDrivenAxle - 2 [Emot1, Emot3+Emot4]

aVarTruthTableCondition_6 = logical(u1 == 1 && u2 == 2);

% 1stDrivenAxle - 2  and 2ndDrivenAxle - 0 [Emot1+Emot2,-]

aVarTruthTableCondition_7 = logical(u1 == 2 && u2 == 0);

% 1stDrivenAxle - 2  and 2ndDrivenAxle - 1 [Emot1+Emot2,Emot3]

aVarTruthTableCondition_8 = logical(u1 == 2 && u2 == 1);

% 1stDrivenAxle - 2  and2ndDrivenAxle - 2 [Emot1+Emot2,Emot3+Emot4]

aVarTruthTableCondition_9 = logical(u1 == 2 && u2 == 2);

if (aVarTruthTableCondition_1 && ~aVarTruthTableCondition_2 && ~aVarTruthTableCondition_3 && ~aVarTruthTableCondition_4 && ~aVarTruthTableCondition_5 && ~aVarTruthTableCondition_6 && ~aVarTruthTableCondition_7 && ~aVarTruthTableCondition_8 && ~aVarTruthTableCondition_9)
    aFcnTruthTableAction_1();
elseif (~aVarTruthTableCondition_1 && aVarTruthTableCondition_2 && ~aVarTruthTableCondition_3 && ~aVarTruthTableCondition_4 && ~aVarTruthTableCondition_5 && ~aVarTruthTableCondition_6 && ~aVarTruthTableCondition_7 && ~aVarTruthTableCondition_8 && ~aVarTruthTableCondition_9)
    aFcnTruthTableAction_2();
elseif (~aVarTruthTableCondition_1 && ~aVarTruthTableCondition_2 && aVarTruthTableCondition_3 && ~aVarTruthTableCondition_4 && ~aVarTruthTableCondition_5 && ~aVarTruthTableCondition_6 && ~aVarTruthTableCondition_7 && ~aVarTruthTableCondition_8 && ~aVarTruthTableCondition_9)
    aFcnTruthTableAction_3();
elseif (~aVarTruthTableCondition_1 && ~aVarTruthTableCondition_2 && ~aVarTruthTableCondition_3 && aVarTruthTableCondition_4 && ~aVarTruthTableCondition_5 && ~aVarTruthTableCondition_6 && ~aVarTruthTableCondition_7 && ~aVarTruthTableCondition_8 && ~aVarTruthTableCondition_9)
    aFcnTruthTableAction_4();
elseif (~aVarTruthTableCondition_1 && ~aVarTruthTableCondition_2 && ~aVarTruthTableCondition_3 && ~aVarTruthTableCondition_4 && aVarTruthTableCondition_5 && ~aVarTruthTableCondition_6 && ~aVarTruthTableCondition_7 && ~aVarTruthTableCondition_8 && ~aVarTruthTableCondition_9)
    aFcnTruthTableAction_5();
elseif (~aVarTruthTableCondition_1 && ~aVarTruthTableCondition_2 && ~aVarTruthTableCondition_3 && ~aVarTruthTableCondition_4 && ~aVarTruthTableCondition_5 && aVarTruthTableCondition_6 && ~aVarTruthTableCondition_7 && ~aVarTruthTableCondition_8 && ~aVarTruthTableCondition_9)
    aFcnTruthTableAction_6();
elseif (~aVarTruthTableCondition_1 && ~aVarTruthTableCondition_2 && ~aVarTruthTableCondition_3 && ~aVarTruthTableCondition_4 && ~aVarTruthTableCondition_5 && ~aVarTruthTableCondition_6 && aVarTruthTableCondition_7 && ~aVarTruthTableCondition_8 && ~aVarTruthTableCondition_9)
    aFcnTruthTableAction_7();
elseif (~aVarTruthTableCondition_1 && ~aVarTruthTableCondition_2 && ~aVarTruthTableCondition_3 && ~aVarTruthTableCondition_4 && ~aVarTruthTableCondition_5 && ~aVarTruthTableCondition_6 && ~aVarTruthTableCondition_7 && aVarTruthTableCondition_8 && ~aVarTruthTableCondition_9)
    aFcnTruthTableAction_8();
elseif (~aVarTruthTableCondition_1 && ~aVarTruthTableCondition_2 && ~aVarTruthTableCondition_3 && ~aVarTruthTableCondition_4 && ~aVarTruthTableCondition_5 && ~aVarTruthTableCondition_6 && ~aVarTruthTableCondition_7 && ~aVarTruthTableCondition_8 && aVarTruthTableCondition_9)
    aFcnTruthTableAction_9();
else % Default
    aFcnTruthTableAction_10();
end

function aFcnTruthTableAction_1()

% 1stDrivenAxle - 0 
% 2ndDrivenAxle - 0
% NOT VALID

y1 = 0;
y2 = 0;
y3 = 0;
y4 = 0;

function aFcnTruthTableAction_2()

% 1stDrivenAxle - 0 
% 2ndDrivenAxle - 1
% NOT VALID

y1 = 0;
y2 = 0;
y3 = 0;
y4 = 0;

function aFcnTruthTableAction_3()

% 1stDrivenAxle - 0 
% 2ndDrivenAxle - 2
% NOT VALID

y1 = 0;
y2 = 0;
y3 = 0;
y4 = 0;

function aFcnTruthTableAction_4()

% 1stDrivenAxle - 1 
% 2ndDrivenAxle - 0 [Emot1,-]

y1 = 1;
y2 = 0;
y3 = 0;
y4 = 0;

function aFcnTruthTableAction_5()

% 1stDrivenAxle - 1  
% 2ndDrivenAxle - 1 [Emot1, Emot3]

y1 = 1;
y2 = 0;
y3 = 1;
y4 = 0;

function aFcnTruthTableAction_6()

% 1stDrivenAxle - 1 
% 2ndDrivenAxle - 2 [Emot1, Emot3+Emot4]

y1 = 1;
y2 = 0;
y3 = 1;
y4 = 1;

function aFcnTruthTableAction_7()

% 1stDrivenAxle - 2  
% 2ndDrivenAxle - 0 [Emot1+Emot2,-]

y1 = 1;
y2 = 1;
y3 = 0;
y4 = 0;

function aFcnTruthTableAction_8()

% 1stDrivenAxle - 2  
% 2ndDrivenAxle - 1 [Emot1+Emot2,Emot3]

y1 = 1;
y2 = 1;
y3 = 1;
y4 = 0;

function aFcnTruthTableAction_9()

% 1stDrivenAxle - 2
% 2ndDrivenAxle - 2 [Emot1+Emot2,Emot3+Emot4]

y1 = 1;
y2 = 1;
y3 = 1;
y4 = 1;

function aFcnTruthTableAction_10()

% Default

y1 = 0;
y2 = 0;
y3 = 0;
y4 = 0;
